simulink model "Simple_MassCT_model"  (R2017b)
settings: Solver=VariableStepAuto  StartTime=0.0  StopTime=100  RelTol=1e-3
values from neighbouring files (symbols this model uses):
  b = 0.19    [parameters.m]
  m = 20    [parameters.m]
settings Model: Creator=cespinos  LastModifiedBy=cespinos

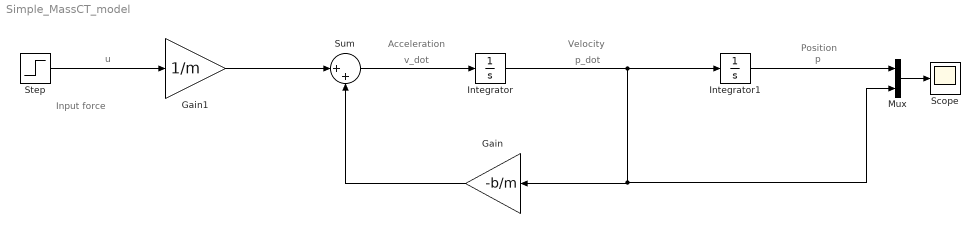
== system Simple_MassCT_model ==
  note: Position
  note: Velocity
  note: Acceleration
  note: Input force
  note: p
  note: u
  note: p_dot
  note: v_dot
  Gain : Gain  Gain=-b/m
  Gain1 : Gain  Gain=1/m
  Integrator : Integrator
  Integrator1 : Integrator
  Mux : Mux  Inputs=2
  Scope : Scope
  Step : Step  After=0.02  SampleTime=0
  Sum : Sum  Inputs=|++
  wires:
  Sum/1 -> Integrator/1
  Integrator/1 -> Mux/2, Gain/1, Integrator1/1
  Gain/1 -> Sum/2
  Gain1/1 -> Sum/1
  Step/1 -> Gain1/1
  Mux/1 -> Scope/1
  Integrator1/1 -> Mux/1
